simulink model "motor_beam_model_sim"  (R2022b)
settings: Solver=VariableStepAuto  StartTime=0.0  StopTime=10.0  MaxStep=5.0E-5  RelTol=1e-3
values from neighbouring files (symbols this model uses):
  A = d_sys.A    [motor_beam_sim_main.m]
  A_augmented = [A zeros(4,1) ... (first row only)    [motor_beam_sim_main.m]
  Ac = [0, 1, 0, 0 ... (first row only)    [motor_beam_sim_main.m]
  B = d_sys.B    [motor_beam_sim_main.m]
  B_augmented = [B ... (first row only)    [motor_beam_sim_main.m]
  Bc = [0 0 0 k_v]'    [motor_beam_sim_main.m]
  C = d_sys.C    [motor_beam_sim_main.m]
  Cs = [-1 -1.5 5 1]    [motor_beam_sim_main.m]
  Cs_integral_action = [-1.3 -1.5 4 1 -0.0019]    [motor_beam_sim_main.m]
  CTLR = 6    [motor_beam_sim_main.m]
  g = 9.81    [motor_beam_sim_main.m]
  gamma = 0.4    [motor_beam_sim_main.m]
  gamma_integral_action = 0.7    [motor_beam_sim_main.m]
  input_limit = [10, -10]    [motor_beam_sim_main.m]
  input_noise = 1    [motor_beam_sim_main.m]
  J_b = 2/5*m*r^2    (= 1.3196e-06)    [motor_beam_sim_main.m]
  K = place(A,B,p_discrete)    [motor_beam_sim_main.m]
  K_sfc_integral_action = place(A_augmented,B_augmented,p_discrete_integral)    [motor_beam_sim_main.m]
  k_theta_dot = -84.45    [motor_beam_sim_main.m]
  k_v = 20.83    [motor_beam_sim_main.m]
  L = place(A',C',po_discrete)'    [motor_beam_sim_main.m]
  m = 0.03299    [motor_beam_sim_main.m]
  OBS = 1    [motor_beam_sim_main.m]
  P_0 = 0*eye(4,4)    [motor_beam_sim_main.m]
  Q = 1e-10* eye(4)    [motor_beam_sim_main.m]
  R = diag([position_variance^2, angle_variance^2])    [motor_beam_sim_main.m]
  r = 0.01    [motor_beam_sim_main.m]
  sensor_noise = 1    [motor_beam_sim_main.m]
  Ts = 1/fs    (= 0.01)    [motor_beam_sim_main.m]
  xo = [0.4 0.0 0.0 0.0]'    [motor_beam_sim_main.m]
  xo_hat = [0.4 0.0 0.0 0.0]'    [motor_beam_sim_main.m]
undefined symbols (not defined in the file or in its folder): Kf, Kf_and_Ki
libraries: dspsrcs4 x3
settings Model: Creator=lucien  LastModifiedBy=lucien
settings DebuggingCC: UnderSpecifiedDimensionMsg=warning

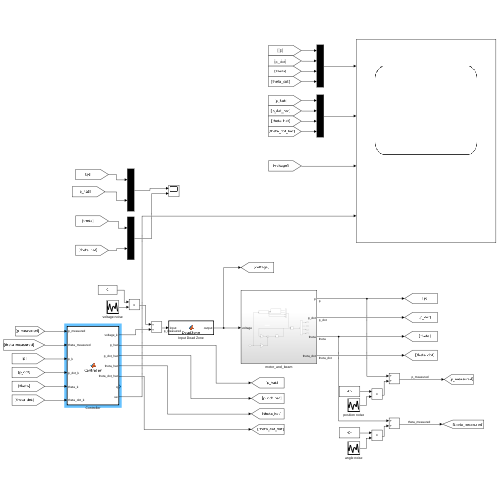
[thumbnail: Simulink's stored preview of the top-level diagram]
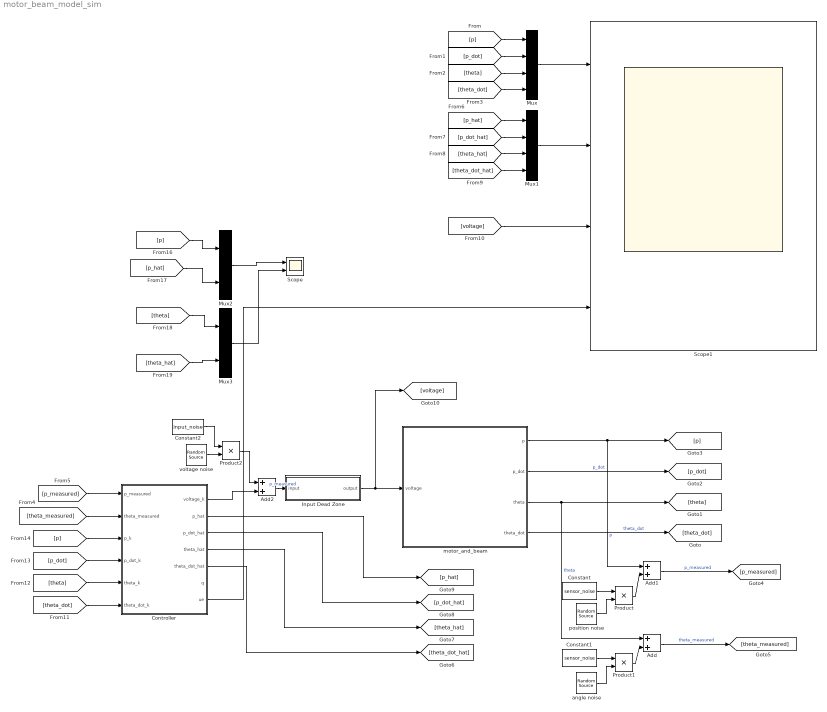
== system motor_beam_model_sim ==
  Add : Sum
  Add1 : Sum
  Add2 : Sum
  Constant : Constant  Value=sensor_noise
  Constant1 : Constant  Value=sensor_noise
  Constant2 : Constant  Value=input_noise
  Controller : MATLAB Function  TreatAsAtomicUnit=on  SystemSampleTime=Ts
  Input Dead Zone : MATLAB Function  TreatAsAtomicUnit=on
  Mux : Mux
  Mux1 : Mux
  Mux2 : Mux  Inputs=2
  Mux3 : Mux  Inputs=2
  Product : Product
  Product1 : Product
  Product2 : Product
  Scope : Scope  NumInputPorts=2
  Scope1 : Scope  NumInputPorts=4
  angle noise : dspsrcs4/Random Source  SrcType=Gaussian  NormMethod=Ziggurat  CltLength=12  MinVal=0  MaxVal=1  MeanVal=0  VarVal=angle_variance  RepMode=Not repeatable  rawSeed=1  IsInherit=off  SampMode=Discrete  SampTime=Ts  SampFrame=1  DataType=Double  OutComplex=Real  OutputFrames=off
  motor_and_beam : Subsystem
  position noise : dspsrcs4/Random Source  SrcType=Gaussian  NormMethod=Ziggurat  CltLength=12  MinVal=0  MaxVal=1  MeanVal=0  VarVal=position_variance  RepMode=Not repeatable  rawSeed=1  IsInherit=off  SampMode=Discrete  SampTime=Ts  SampFrame=1  DataType=Double  OutComplex=Real  OutputFrames=off
  voltage noise : dspsrcs4/Random Source  SrcType=Gaussian  NormMethod=Ziggurat  CltLength=12  MinVal=0  MaxVal=1  MeanVal=0  VarVal=voltage_noise  RepMode=Not repeatable  rawSeed=1  IsInherit=off  SampMode=Discrete  SampTime=Ts  SampFrame=1  DataType=Double  OutComplex=Real  OutputFrames=off
  wires:
  motor_and_beam/1(p) -> Add1/1, [p]  "p"
  motor_and_beam/3(theta) -> Add/1, [theta]  "theta"
  Add1/1 -> [p_measured]  "p_measured"
  Add/1 -> [theta_measured]  "theta_measured"
  [theta_measured] -> Controller/2(theta_measured)
  [p_measured] -> Controller/1(p_measured)
  Controller/2(p_hat) -> [p_hat]
  Controller/3(p_dot_hat) -> [p_dot_hat]
  Controller/4(theta_hat) -> [theta_hat]
  Controller/5(theta_dot_hat) -> [theta_dot_hat]
  motor_and_beam/2(p_dot) -> [p_dot]  "p_dot"
  motor_and_beam/4(theta_dot) -> [theta_dot]  "theta_dot"
  [p] -> Mux/1
  [p_dot] -> Mux/2
  [theta] -> Mux/3
  [theta_dot] -> Mux/4
  [p_hat] -> Mux1/1
  [p_dot_hat] -> Mux1/2
  [theta_hat] -> Mux1/3
  [theta_dot_hat] -> Mux1/4
  [voltage] -> Scope1/3
  Mux/1 -> Scope1/1
  Mux1/1 -> Scope1/2
  [p] -> Mux2/1
  [p_hat] -> Mux2/2
  Mux2/1 -> Scope/1
  [theta] -> Mux3/1
  [theta_hat] -> Mux3/2
  Mux3/1 -> Scope/2
  Input Dead Zone/1(output) -> [voltage], motor_and_beam/1(voltage)
  position noise/1 -> Product/2
  Product/1 -> Add1/2
  Constant/1 -> Product/1
  Product1/1 -> Add/2
  angle noise/1 -> Product1/2
  Constant1/1 -> Product1/1
  Constant2/1 -> Product2/1
  voltage noise/1 -> Product2/2
  Add2/1 -> Input Dead Zone/1(input)  "p_measured"
  Controller/1(voltage_k) -> Add2/2
  Product2/1 -> Add2/1
  [theta_dot] -> Controller/6(theta_dot_k)
  [theta] -> Controller/5(theta_k)
  [p_dot] -> Controller/4(p_dot_k)
  [p] -> Controller/3(p_k)
  Controller/7(ue) -> Scope1/4

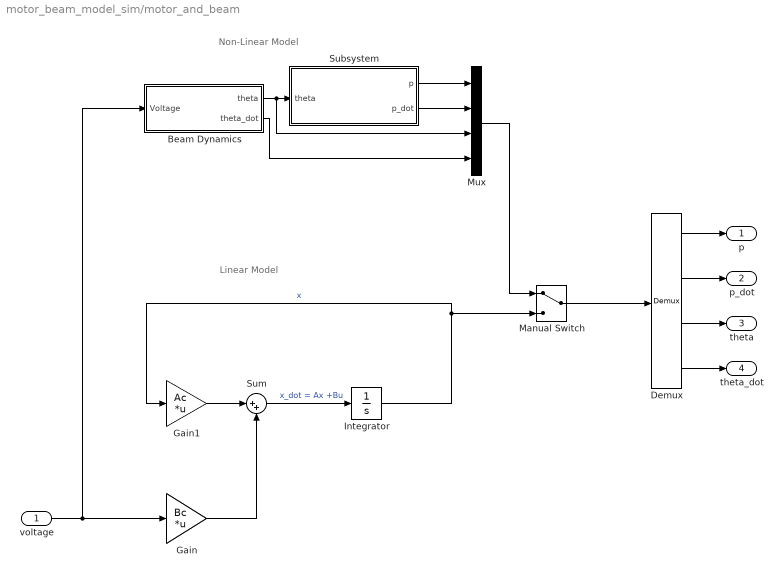
== system motor_beam_model_sim/motor_and_beam ==
  note: Non-Linear Model
  note: Linear Model
  voltage : Inport
  Beam Dynamics : Subsystem
  Demux : Demux
  Gain : Gain  Gain=Bc  Multiplication=Matrix(K*u)
  Gain1 : Gain  Gain=Ac  Multiplication=Matrix(K*u)
  Integrator : Integrator  InitialCondition=xo
  Manual Switch : ManualSwitch
  Mux : Mux
  Subsystem : Subsystem
  Sum : Sum  Inputs=|++
  p : Outport
  p_dot : Outport  Port=2
  theta : Outport  Port=3
  theta_dot : Outport  Port=4
  wires:
  voltage/1 -> Beam Dynamics/1(Voltage), Gain/1
  Gain/1 -> Sum/2
  Sum/1 -> Integrator/1  "x_dot = Ax +Bu"
  Gain1/1 -> Sum/1
  Integrator/1 -> Manual Switch/2, Gain1/1  "x"
  Demux/4 -> theta_dot/1
  Demux/3 -> theta/1
  Demux/2 -> p_dot/1
  Demux/1 -> p/1
  Manual Switch/1 -> Demux/1
  Beam Dynamics/1(theta) -> Mux/3, Subsystem/1(theta)
  Subsystem/1(p) -> Mux/1
  Subsystem/2(p_dot) -> Mux/2
  Beam Dynamics/2(theta_dot) -> Mux/4
  Mux/1 -> Manual Switch/1

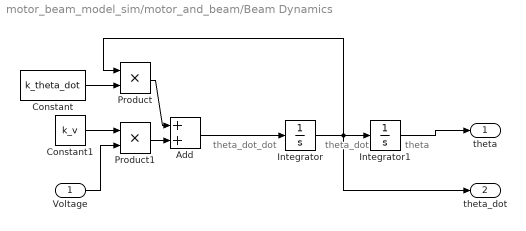
== system motor_beam_model_sim/motor_and_beam/Beam Dynamics ==
  note: theta
  note: theta_dot
  note: theta_dot_dot
  Voltage : Inport
  Add : Sum
  Constant : Constant  Value=k_theta_dot
  Constant1 : Constant  Value=k_v
  Integrator : Integrator  InitialCondition=xo(4)
  Integrator1 : Integrator  InitialCondition=xo(3)
  Product : Product
  Product1 : Product
  theta : Outport
  theta_dot : Outport  Port=2
  wires:
  Voltage/1 -> Product1/2
  Constant/1 -> Product/2
  Product1/1 -> Add/2
  Constant1/1 -> Product1/1
  Integrator/1 -> theta_dot/1, Product/1, Integrator1/1
  Add/1 -> Integrator/1
  Integrator1/1 -> theta/1
  Product/1 -> Add/1

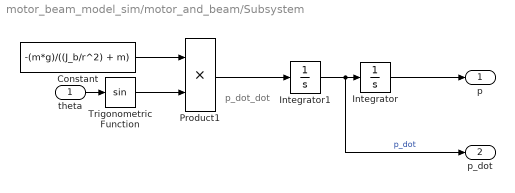
== system motor_beam_model_sim/motor_and_beam/Subsystem ==
  note: p_dot_dot
  theta : Inport
  Constant : Constant  Value=-(m*g)/((J_b/r^2) + m)
  Integrator : Integrator  InitialCondition=xo(1)
  Integrator1 : Integrator  InitialCondition=xo(2)
  Product1 : Product
  Trigonometric Function : Trigonometry
  p : Outport
  p_dot : Outport  Port=2
  wires:
  theta/1 -> Trigonometric Function/1
  Trigonometric Function/1 -> Product1/2
  Constant/1 -> Product1/1
  Product1/1 -> Integrator1/1
  Integrator1/1 -> p_dot/1, Integrator/1  "p_dot"
  Integrator/1 -> p/1

== matlab function motor_beam_model_sim/Input Dead Zone ==
  settings: updateMethod=CONTINUOUS  sampleTime=Ts
  data: input input; output output; dead_zone parameter
function output  = DeadZone(input, dead_zone)

if(input > dead_zone(1)) || (input < dead_zone(2))
    output = input;
else
    output = 0;
end
end

== matlab function motor_beam_model_sim/Controller ==
  settings: updateMethod=DISCRETE  sampleTime=Ts
  data: p_measured input; theta_measured input; p_k input; p_dot_k input; theta_k input; theta_dot_k input; xo_hat parameter; OBS parameter; CTLR parameter; input_limit parameter; A parameter; B parameter; C parameter; K parameter; L parameter; voltage_k output size=1; p_hat output size=1; p_dot_hat output size=1; theta_hat output size=1; theta_dot_hat output size=1; Q parameter; R parameter; P_0 parameter; Kf parameter; q output; Kf_and_Ki parameter; Cs parameter; gamma parameter; K_sfc_integral_action parameter; Cs_integral_action parameter; gamma_integral_action parameter; ue output; A_augmented parameter; B_augmented parameter
function [voltage_k, p_hat, p_dot_hat, theta_hat, theta_dot_hat,q,ue] = Controller(p_measured, theta_measured, p_k, p_dot_k, theta_k, theta_dot_k, xo_hat, OBS, CTLR, input_limit, A, B, C, K, L, Q, R, P_0, Kf, Kf_and_Ki,Cs, gamma,K_sfc_integral_action,Cs_integral_action,gamma_integral_action,A_augmented, B_augmented)
%% Initialise system and covaraince on first call
persistent x_hat_k
if isempty(x_hat_k)
    x_hat_k = xo_hat; %observer initialization x_hat(0) 
end

persistent P_k
if isempty(P_k)
    P_k = P_0; % Kalman Filter parameter
end

persistent q_k
if isempty(q_k)
    q_k = 0; % integral action parameter
end

persistent u_e
if isempty(u_e)
    u_e = 0; % integral action parameter
end
%% Control
% Desired setpoint
x_ref = [-0.2, 0, 0, 0]';
% Desired reference to hold the setpoint
u_ref=0;

% check if observer is required
if (OBS == 0)
    x_k = [p_k, p_dot_k, theta_k, theta_dot_k]';
else
    x_k = x_hat_k;
end

% calculate control action
if (CTLR == 1)% SFC
    voltage_k=-K*(x_k-x_ref)+u_ref;
elseif(CTLR == 2) % SFC + integral action
    %update q_k (position error integration)
    q_k = q_k + x_k(1) - x_ref(1);
    x_e = [(x_k-x_ref); q_k];
    voltage_k=-K_sfc_integral_action*x_e+u_ref;
elseif (CTLR == 3) % LQR
    voltage_k=-Kf*(x_k-x_ref)+u_ref;
elseif (CTLR == 4) % LQR + integral action
    %update q_k (position error integration)
    q_k = q_k + x_k(1) - x_ref(1);
    x_e = [(x_k-x_ref); q_k];
    voltage_k=-Kf_and_Ki*x_e+u_ref;
elseif(CTLR == 5) % SMC
    xe = x_k - x_ref;
    Sx=Cs*xe;                        %surface
    Keq=inv(Cs*B)*Cs*A;          %Equivalent feedback matrix
    ueq=-Keq*xe;                     %Equivalent Input
    usw=-inv(Cs*B)*gamma*tanh(Sx);  %Switching Input
    voltage_k=ueq+usw;                    %SMC input
elseif(CTLR == 6) % SMC + integral action
    %update q_k (position error integration)
    q_k = q_k + x_k(1) - x_ref(1);
    x_e = [(x_k-x_ref); q_k];
    Sx=Cs_integral_action*x_e;    %surface
    Keq=inv(Cs_integral_action*B_augmented)*Cs_integral_action*A_augmented;          %Equivalent feedback matrix
    ueq=-Keq*x_e;                     %Equivalent Input
    usw=-inv(Cs_integral_action*B_augmented)*gamma_integral_action*tanh(Sx);  %Switching Input
    voltage_k=ueq+usw;                    %SMC input
    u_e = ueq;
else % assume open loop
    voltage_k = 0;
end

% input limits
voltage_k = min(voltage_k, input_limit(1));
voltage_k = max(voltage_k, input_limit(2));


%% Observers
% construct the measurement vector
z_k = [p_measured, theta_measured]';

if(CTLR == 1)||(CTLR == 2) % Luenberger
    x_hat_k = A * x_hat_k + B * voltage_k +L * (z_k - C*x_hat_k);

elseif (CTLR == 3)||(CTLR == 4)||(CTLR == 5)||(CTLR == 6) % Kalman Filter
    % predict
    % predict state forward
    x_hat_k_plus_1_priori = A * x_hat_k + B * voltage_k;
    % predict covaraince forward
    P_k_plus_1_priori = A * P_k * A' + Q;
    
    % update
    % compute kalman gain
    k_gain = P_k_plus_1_priori * C' / (C*P_k_plus_1_priori*C'+R);
    % predict measurement for predicted state
    measurement_predict = C * x_hat_k_plus_1_priori;
    % update and correct estimate for x_hat
    innovation = z_k - measurement_predict;
    x_hat_k_plus_1 = x_hat_k_plus_1_priori + k_gain*(innovation);
    % update and correct estimate for covariance
    P_k = (eye(4,4) - k_gain * C) * P_k_plus_1_priori;
    x_hat_k = A * x_hat_k + B * voltage_k + k_gain * innovation;
else
    x_hat_k = xo_hat;
end

%% Output current estimates
p_hat = x_hat_k(1);
p_dot_hat = x_hat_k(2);
theta_hat = x_hat_k(3);
theta_dot_hat = x_hat_k(4);
q = q_k;
ue = u_e;
end
